simulink model "Pdot_test"  (R2016b)
settings: Solver=VariableStepAuto  StartTime=0.0  StopTime=10.0  RelTol=1e-3
undefined symbols (not defined in the file or in its folder): DiscIntNeverNeededParam
settings Model: Creator=root  LastModifiedBy=root

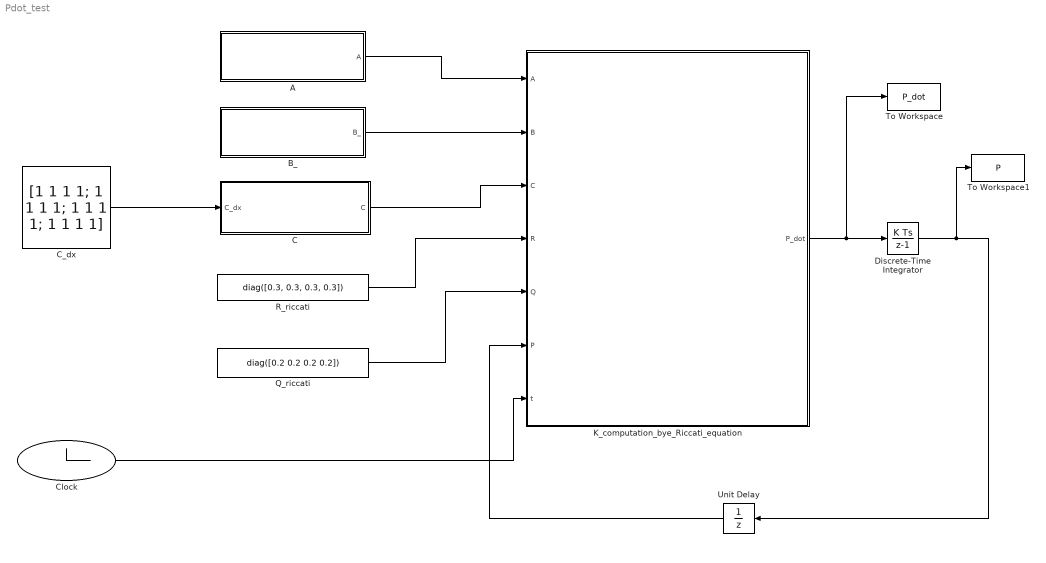
== system Pdot_test ==
  A : MATLAB Function  TreatAsAtomicUnit=on
  B_ : MATLAB Function  TreatAsAtomicUnit=on
  C : MATLAB Function  TreatAsAtomicUnit=on
  C_dx : Constant  Value=[1 1 1 1; 1 1 1 1; 1 1 1 1; 1 1 1 1]
  Clock : Clock
      settings: Decimation=50
  Discrete-Time Integrator : DiscreteIntegrator  InitialConditionSetting=State (most efficient)  SampleTime=-1  ICPrevOutput=DiscIntNeverNeededParam  ICPrevScaledInput=DiscIntNeverNeededParam
  K_computation_bye_Riccati_equation : MATLAB Function  TreatAsAtomicUnit=on
  Q_riccati : Constant  Value=diag([0.2 0.2 0.2 0.2])
  R_riccati : Constant  Value=diag([0.3, 0.3, 0.3, 0.3])
  To Workspace : ToWorkspace  VariableName=P_dot  SampleTime=-1
  To Workspace1 : ToWorkspace  VariableName=P  SampleTime=-1
  Unit Delay : UnitDelay  SampleTime=-1
  wires:
  C_dx/1 -> C/1(C_dx)
  R_riccati/1 -> K_computation_bye_Riccati_equation/4(R)
  A/1(A) -> K_computation_bye_Riccati_equation/1(A)
  Q_riccati/1 -> K_computation_bye_Riccati_equation/5(Q)
  C/1(C) -> K_computation_bye_Riccati_equation/3(C)
  B_/1(B_) -> K_computation_bye_Riccati_equation/2(B)
  K_computation_bye_Riccati_equation/1(P_dot) -> To Workspace/1, Discrete-Time Integrator/1
  Discrete-Time Integrator/1 -> To Workspace1/1, Unit Delay/1
  Unit Delay/1 -> K_computation_bye_Riccati_equation/6(P)
  Clock/1 -> K_computation_bye_Riccati_equation/7(t)

== matlab function Pdot_test/B_ ==
  data: B_ output
function B_ = B()

 B_ = zeros(10,3);

 B_(8:10,1:3) = eye(3);
end

== matlab function Pdot_test/K_computation_bye_Riccati_equation ==
  data: A input; B input; C input; R input; Q input; P input size=[10,10]; t input; P_dot output
function P_dot  = P_dot_func(A,B,C,R,Q,P,t)

%K = zeros(10,3);
if (t == 0)
   
   P = diag([3*10^3, 3*10^3, 3*10^3, 3*10^3, 10, 10, 10, 0.01, 0.01, 0.01]);
   % P = diag([1,1,1,1,1,1,1,1,1,1]);
    %P = zeros(10);
   
end

%coder.extrinsic('are');

%Q_ = C'*C;

%[P,L,G] = care(A,C',Q_,R);

R_inv = pinv(R); 

P_dot = P*A + A'*P - P*C'*R_inv*C*P + C'*C;

%P = are(A, C'*R_inv*C, C);

%K = P*C'*R_inv;

end

== matlab function Pdot_test/A ==
  data: A output
function A = A()

 A = zeros(10);

 A(1:3,5:7) = eye(3);
 A(5:7,8:10) = eye(3);
 
end

== matlab function Pdot_test/C ==
  data: C output; C_dx input
function C = C(C_dx)

   row = size(C_dx,1); 

   C1 = zeros(row,6);

 C = [2*C_dx C1];
 
end
